simulink model "tqdtqr_rebuild_V3"  (R2021b)
settings: Solver=VariableStepAuto  StartTime=0.0  StopTime=10.0  RelTol=1e-3
undefined symbols (not defined in the file): ATQD_AfterTqMinGain_X_Deg, ATQD_APSCreepBaseTqD_X_kph, ATQD_APSCreepBaseTqD_Y_Deg, ATQD_APSCreepBaseTqR_X_kph, ATQD_APSCreepBaseTqR_Y_Deg, ATQD_APSCreepIterm_X_kph, ATQD_APSCreepIterm_Y_kph, ATQD_APSCreepPterm_X_kph, ATQD_APSCreepPterm_Y_kph, ATQD_APSDecReq_X_kph, ATQD_APSDecReq_Y_mps2, ATQD_APSDecReqCMD_X_kph, ATQD_APSDecReqTs_X_pct, ATQD_APSDecTimeGain_X_Deg, ATQD_APSDecTimeGain_Y_s, ATQD_APSReqLowSpd_X_Deg, ATQD_AutoHoldReleaseBPS_X_Deg, ATQD_AWDLoadTrqnsGain_X_kg, ATQD_AWDLoadTrqnsGain_Y_pct, ATQD_BOSEnBPSPosn_X_kph, ATQD_BOSMap_X_rpm, ATQD_BOSMap_Y_pct, ATQD_CreepBaseTqD_X_kph, ATQD_CreepBaseTqD_Y_Deg, ATQD_CreepBaseTqR_X_kph, ATQD_CreepBaseTqR_Y_Deg, ATQD_CreepBPSDisPosn_X_Deg, ATQD_CreepBPSDisPosnR_X_Deg, ATQD_CreepBPSEnPosn_X_Deg, ATQD_CreepBPSEnPosnR_X_Deg, ATQD_CreepDeltaTq_X_kph, ATQD_CreepIterm_X_kph, ATQD_CreepIterm_Y_kph, ATQD_CreepItermMaxLimit_X_pct, ATQD_CreepPreloadTime_X_kph, ATQD_CreepPreloadTq_X_kph, ATQD_CreepPreloadTq_Y_s, ATQD_CreepProtTq_X_Deg, ATQD_CreepPterm_X_kph, ATQD_CreepPterm_Y_kph, ATQD_CreepRrTqSpRat_X_rpm, ATQD_CreepRrTqSpRat_Y_Nm, ATQD_CreepTargetSpdD_X_pct, ATQD_CreepTargetSpdR_X_pct, ATQD_CreepUpLimitTq_X_rpm, ATQD_DecIneOPDHoldEnDelay_X_Deg, ATQD_DecIneOPDHoldEnDelay_Y_bar, ATQD_ECOTqMapD_X_rpm, ATQD_ECOTqMapD_Y_pct, ATQD_EMTqMapD_X_rpm, ATQD_EMTqMapD_Y_pct, ATQD_EOPDTqMapDCon_X_rpm, ATQD_EOPDTqMapDCon_Y_Deg, ATQD_EstInitVehWeight_X_c, ATQD_FAfterTqCMDGain_X_rpm, ATQD_FAfterTqCMDGain_Y_pct, ATQD_ForceLowSpd_X_Deg, ATQD_ForcePLimitSpd_X_Deg, ATQD_FrLossMAPLowV_X_rpm, ATQD_FrLossMAPLowV_Y_Nm ... (+949)
libraries: simulink x235, hcu_lib x208, tqr x63, tqd x6
(part 37 of 37)

== stateflow chart tqdtqr_rebuild_V3/Input_Convert/Signal function/SWC1 SWC2 status/SWC_Subsystem/Speed Setting Mode/ACC Speed Setting ON/ACCSetSpd_Chart_W ==
  state ACCSetSpeed_W
    (default) -> (junction 431) : {VTQD_ACCSetSpd_kph = ZERO_FLOAT;
        |  VTQD_ACCSavedSetSpd_kph = ZERO_FLOAT;
        |  VTQD_UpDownDetCount_sec = ZERO_FLOAT;
        |  VTQD_StandbyOvrdDetEnd_flg = FALSE;}
    ACCSetSpeed_W -> (junction 538) [order 3]
    (junction 538) -> (junction 552) [order 1] : [VTQD_DistanceUnit_flg == VINP_Distanceunit_flg || VTQD_ACCSavedSetSpd_kph <= ONE_FLOAT]
    (junction 552) -> (junction 431) : {VTQD_ACCSetSpd_kph = min(KTQD_ACCActiveMetSpdHi_raw32, VTQD_ACCSavedSetSpd_kph);
        |  VTQD_ACCSavedSetSpd_kph = VTQD_ACCSetSpd_kph;}
    (junction 538) -> (junction 540) [order 2]
    (junction 550) -> (junction 552)
    (junction 431) -> (junction 432) : {VSCP_ActiveDown_flg = FALSE;
        |  VTQD_ActiveUp_flg = FALSE;
        |  VTQD_UpDownTimeCount_sec = ZERO_FLOAT;}
    (junction 540) -> (junction 542) [order 1] : [VINP_Distanceunit_flg == TRUE]
    (junction 540) -> (junction 636) [order 2] : {VTQD_ACCSavedSetSpd_kph = (VTQD_ACCSavedSetSpd_kph * MPH2KPH)}
    (junction 542) -> (junction 599) : {VTQD_ACCSavedSetSpd_kph = (VTQD_ACCSavedSetSpd_kph * KPH2MPH)}
    (junction 432) -> (junction 530) [order 1] : [VINP_ADASACCSta_enum == ENUM_ADASACCSTA_STANDBY ||...
        |  VINP_ADASACCSta_enum == ENUM_ADASACCSTA_OVERRIDE]
    (junction 530) -> (junction 433) [order 1] : [VTQD_SWCSetDownSta_flg == TRUE ||...
        |  VTQD_SWCResUpSta_flg == TRUE]
    (junction 433) -> (junction 419) [order 1] : [VTQD_SWCSetDownSta_flg == TRUE &&...
        |  VTQD_StandbyOvrdDetEnd_flg == FALSE &&...
        |  VTQD_AllowSetSpd_flg == TRUE]
    (junction 432) -> (junction 403) [order 2]
    (junction 530) -> (junction 533) [order 2] : {VTQD_StandbyOvrdDetEnd_flg = FALSE;
        |  VTQD_ACCSetSpd_kph = VTQD_ACCSavedSetSpd_kph;
        |  VTQD_ACCSavedSetSpd_kph = VTQD_ACCSetSpd_kph;
        |  VTQD_DistanceUnit_flg = VINP_Distanceunit_flg;}
    (junction 433) -> (junction 490) [order 2]
    (junction 419) -> (junction 408) : {VTQD_UpDownDetCount_sec = VTQD_UpDownDetCount_sec + task_time_s;}
    (junction 599) -> (junction 602) [order 1] : [VTQD_ACCSavedSetSpd_kph < KTQD_ACCActiveMetSpdLoMPH_mph]
    (junction 636) -> (junction 623) [order 1] : [VTQD_ACCSavedSetSpd_kph < KTQD_ACCActiveMetSpdLo_kph]
    (junction 602) -> (junction 604) : {VTQD_ACCSavedSetSpd_kph = KTQD_ACCActiveMetSpdLoMPH_mph}
    (junction 636) -> (junction 633) [order 2]
    (junction 623) -> (junction 619) : {VTQD_ACCSavedSetSpd_kph = KTQD_ACCActiveMetSpdLo_kph}
    (junction 599) -> (junction 606) [order 2]
    (junction 604) -> (junction 606)
    (junction 619) -> (junction 633)
    (junction 606) -> (junction 613)
    (junction 633) -> (junction 630)
    (junction 630) -> (junction 625) [order 1] : [VTQD_ACCSavedSetSpd_kph > KTQD_ACCActiveMetSpdHi_kph]
    (junction 613) -> (junction 608) [order 1] : [VTQD_ACCSavedSetSpd_kph > KTQD_ACCActiveMetSpdHiMPH_mph]
    (junction 403) -> (junction 395) [order 1] : [(VTQD_SWCSetDownSta_flg == TRUE ||...
        |   VTQD_SWCResUpSta_flg == TRUE) &&...
        |  (VTQD_StandbyOvrdDetEnd_flg == TRUE ||...
        |   VTQD_HoldResDet_flg == TRUE)]
    (junction 490) -> (junction 492) [order 1] : [VINP_ADASACCSta_enum == ENUM_ADASACCSTA_STANDBY &&...
        |  VTQD_SWCResUpSta_flg == TRUE &&...
        |  VTQD_ACCSavedSetSpd_kph > ZERO_FLOAT]
    (junction 408) -> (junction 409) [order 1] : [VTQD_UpDownDetCount_sec > ZERO_FLOAT]
    (junction 409) -> (junction 405) [order 1] : [KTQD_ACCActiveMetSpdHi_raw32 >= VVMC_MeterIndSpeed_raw32 &&...
        |  VVMC_MeterIndSpeed_raw32 >= KTQD_ACCActiveMetSpdLo_raw32]
    (junction 630) -> (junction 632) [order 2]
    (junction 625) -> (junction 628) : {VTQD_ACCSavedSetSpd_kph = KTQD_ACCActiveMetSpdHi_kph}
    (junction 613) -> (junction 615) [order 2]
    (junction 608) -> (junction 612) : {VTQD_ACCSavedSetSpd_kph = KTQD_ACCActiveMetSpdHiMPH_mph}
    (junction 403) -> (junction 396) [order 2] : {VTQD_StandbyOvrdDetEnd_flg = FALSE;
        |  VTQD_HoldResDet_flg = FALSE;}
    (junction 395) -> (junction 399) : {VTQD_StandbyOvrdDetEnd_flg = TRUE;
        |  VTQD_HoldResDet_flg = TRUE;}
    (junction 490) -> (junction 496) [order 2]
    (junction 492) -> (junction 494) : {VTQD_StandbyOvrdDetEnd_flg = TRUE}
    (junction 408) -> (junction 436) [order 2] : {VTQD_ACCSetSpd_kph = VTQD_ACCSavedSetSpd_kph;
        |  VTQD_ACCSavedSetSpd_kph = VTQD_ACCSetSpd_kph;
        |  VTQD_DistanceUnit_flg = VINP_Distanceunit_flg;}
    (junction 409) -> (junction 410) [order 2]
    (junction 405) -> (junction 435) : {VTQD_ACCSetSpd_kph = VVMC_MeterIndSpeed_raw32;
        |  VTQD_ACCSavedSetSpd_kph = VTQD_ACCSetSpd_kph;
        |  VTQD_StandbyOvrdDetEnd_flg = TRUE;
        |  VTQD_UpDownDetCount_sec = ZERO_FLOAT;
        |  VTQD_DistanceUnit_flg = VINP_Distanceunit_flg;}
    (junction 628) -> (junction 632)
    (junction 612) -> (junction 615)
    (junction 632) -> (junction 547)
    (junction 615) -> (junction 544)
    (junction 547) -> (junction 544)
    (junction 544) -> (junction 550)
    (junction 494) -> (junction 496)
    (junction 410) -> (junction 429) [order 1] : [KTQD_ACCActiveMetSpdHi_raw32 < VVMC_MeterIndSpeed_raw32]
    (junction 496) -> (junction 407) : {VTQD_ACCSetSpd_kph = VTQD_ACCSavedSetSpd_kph;
        |  VTQD_ACCSavedSetSpd_kph = VTQD_ACCSetSpd_kph;
        |  VTQD_DistanceUnit_flg = VINP_Distanceunit_flg;}
    (junction 410) -> (junction 420) [order 2] : {VTQD_ACCSetSpd_kph = KTQD_ACCActiveMetSpdLo_raw32;
        |  VTQD_ACCSavedSetSpd_kph = VTQD_ACCSetSpd_kph;
        |  VTQD_StandbyOvrdDetEnd_flg = TRUE;
        |  VTQD_UpDownDetCount_sec = ZERO_FLOAT;
        |  VTQD_DistanceUnit_flg = VINP_Distanceunit_flg;}
    (junction 429) -> (junction 430) : {VTQD_ACCSetSpd_kph = KTQD_ACCActiveMetSpdHi_raw32;
        |  VTQD_ACCSavedSetSpd_kph = VTQD_ACCSetSpd_kph;
        |  VTQD_StandbyOvrdDetEnd_flg = TRUE;
        |  VTQD_UpDownDetCount_sec = ZERO_FLOAT;
        |  VTQD_DistanceUnit_flg = VINP_Distanceunit_flg;}
    (junction 399) -> (junction 396)
    (junction 396) -> (junction 438)
    (junction 438) -> (junction 417) [order 1] : [VINP_ADASACCSta_enum == ENUM_ADASACCSTA_ACTIVE]
    (junction 417) -> (junction 434) [order 1] : [VTQD_SWCSetDownSta_flg == TRUE &&...
        |  VTQD_StandbyOvrdDetEnd_flg == FALSE &&...
        |  VVMC_LVDAACCStatusInformation_flg == FALSE]
    (junction 438) -> (junction 427) [order 2]
    (junction 417) -> (junction 412) [order 2]
    (junction 434) -> (junction 411) : {VTQD_UpDownDetCount_sec = VTQD_UpDownDetCount_sec + task_time_s;}
    (junction 411) -> (junction 437) [order 1] : [VTQD_UpDownDetCount_sec > ZERO_FLOAT]
    (junction 411) -> (junction 406) [order 2] : {VTQD_ACCSetSpd_kph = VTQD_ACCSavedSetSpd_kph;
        |  VTQD_ACCSavedSetSpd_kph = VTQD_ACCSetSpd_kph;
        |  VTQD_DistanceUnit_flg = VINP_Distanceunit_flg;}
    (junction 437) -> (junction 428) : {VTQD_ACCSetSpd_kph = max(KTQD_ACCActiveMetSpdLo_raw32, VTQD_ACCSavedSetSpd_kph - ONE_FLOAT);
        |  VTQD_ACCSavedSetSpd_kph = VTQD_ACCSetSpd_kph;
        |  VSCP_ActiveDown_flg = TRUE;
        |  VTQD_UpDownDetCount_sec = ZERO_FLOAT;
        |  VTQD_UpDownTimeCount_sec = task_time_s;
        |  VTQD_DistanceUnit_flg = VINP_Distanceunit_flg;}
    (junction 427) -> (junction 404) [order 1] : [VINP_ADASACCSta_enum == ENUM_ADASACCSTA_OFF ||...
        |  VINP_ADASACCSta_enum == ENUM_ADASACCSTA_DISABLE||...
        |  VINP_ADASACCSta_enum == ENUM_ADASACCSTA_ERROR]
    (junction 412) -> (junction 510) [order 1] : [VTQD_SWCResUpSta_flg == TRUE]
    (junction 510) -> (junction 413) [order 1] : [VTQD_StandbyOvrdDetEnd_flg == FALSE &&...
        |  VVMC_LVDAACCStatusInformation_flg == FALSE &&...
        |  VTQD_HoldResDet_flg == FALSE]
    (junction 427) -> (junction 422) [order 2] : {VTQD_ACCSetSpd_kph = VTQD_ACCSavedSetSpd_kph;
        |  VTQD_ACCSavedSetSpd_kph = VTQD_ACCSetSpd_kph;
        |  VTQD_DistanceUnit_flg = VINP_Distanceunit_flg;}
    (junction 404) -> (junction 426) : {VTQD_ACCSetSpd_kph = ZERO_FLOAT;
        |  VTQD_ACCSavedSetSpd_kph = VTQD_ACCSetSpd_kph;
        |  VTQD_DistanceUnit_flg = VINP_Distanceunit_flg;}
    (junction 412) -> (junction 522) [order 2]
    (junction 510) -> (junction 512) [order 2]
    (junction 413) -> (junction 414) : {VTQD_UpDownDetCount_sec = VTQD_UpDownDetCount_sec + task_time_s;}
    (junction 512) -> (junction 514) [order 1] : [VTQD_StandbyOvrdDetEnd_flg == FALSE &&...
        |  VVMC_LVDAACCStatusInformation_flg != FALSE]
    (junction 414) -> (junction 415) [order 1] : [VTQD_UpDownDetCount_sec > ZERO_FLOAT]
    (junction 512) -> (junction 519) [order 2]
    (junction 514) -> (junction 516) : {VTQD_HoldResDet_flg = TRUE}
    (junction 414) -> (junction 418) [order 2] : {VTQD_ACCSetSpd_kph = VTQD_ACCSavedSetSpd_kph;
        |  VTQD_ACCSavedSetSpd_kph = VTQD_ACCSetSpd_kph;
        |  VTQD_DistanceUnit_flg = VINP_Distanceunit_flg;}
    (junction 415) -> (junction 421) : {VTQD_ACCSetSpd_kph = min(KTQD_ACCActiveMetSpdHi_raw32, VTQD_ACCSavedSetSpd_kph + ONE_FLOAT);
        |  VTQD_ACCSavedSetSpd_kph = VTQD_ACCSetSpd_kph;
        |  VTQD_ActiveUp_flg = TRUE;
        |  VTQD_UpDownDetCount_sec = ZERO_FLOAT;
        |  VTQD_UpDownTimeCount_sec = task_time_s;
        |  VTQD_DistanceUnit_flg = VINP_Distanceunit_flg;}
    (junction 519) -> (junction 522)
    (junction 516) -> (junction 519)
    (junction 522) -> (junction 416) : {VTQD_ACCSetSpd_kph = VTQD_ACCSavedSetSpd_kph;
        |  VTQD_ACCSavedSetSpd_kph = VTQD_ACCSetSpd_kph;
        |  VTQD_DistanceUnit_flg = VINP_Distanceunit_flg;}
    ACCSetSpeed_W -> (junction 568) [order 1] : [VSCP_ActiveDown_flg == TRUE &&...
        |  VINP_ADASACCSta_enum == ENUM_ADASACCSTA_ACTIVE &&...
        |  VTQD_SWCSetDownSta_flg == TRUE]
    (junction 568) -> (junction 556) [order 1] : [VTQD_DistanceUnit_flg == VINP_Distanceunit_flg]
    (junction 556) -> (junction 423)
    (junction 568) -> (junction 558) [order 2]
    (junction 560) -> (junction 556)
    (junction 423) -> (junction 424) : {VTQD_UpDownTimeCount_sec = VTQD_UpDownTimeCount_sec + task_time_s}
    (junction 558) -> (junction 566) [order 1] : [VINP_Distanceunit_flg == TRUE]
    (junction 558) -> (junction 571) [order 2] : {VTQD_ACCSavedSetSpd_kph = (VTQD_ACCSavedSetSpd_kph * MPH2KPH)}
    (junction 566) -> (junction 557) : {VTQD_ACCSavedSetSpd_kph = (VTQD_ACCSavedSetSpd_kph * KPH2MPH)}
    (junction 424) -> (junction 466) [order 1] : [VTQD_UpDownTimeCount_sec >= KTQD_SetSpdLongPLim_s]
    (junction 424) -> (junction 444) [order 2] : {VTQD_ACCSetSpd_kph = VTQD_ACCSavedSetSpd_kph;
        |  VTQD_ACCSavedSetSpd_kph = VTQD_ACCSetSpd_kph;
        |  VTQD_DistanceUnit_flg = VINP_Distanceunit_flg;}
    (junction 466) -> (junction 478) : {VTQD_ACCSetSpd_kph = max(KTQD_ACCActiveMetSpdLo_raw32, ceil(VTQD_ACCSavedSetSpd_kph / KTQD_SetSpdDeltaLong_kph - ONE_FLOAT) * KTQD_SetSpdDeltaLong_kph);
        |  VTQD_ACCSavedSetSpd_kph = VTQD_ACCSetSpd_kph;
        |  VTQD_UpDownTimeCount_sec = ZERO_FLOAT;
        |  VTQD_DistanceUnit_flg = VINP_Distanceunit_flg;}
    (junction 571) -> (junction 557)
    (junction 557) -> (junction 560)
    ACCSetSpeed_W -> (junction 585) [order 2] : [VTQD_ActiveUp_flg == TRUE &&...
        |  VINP_ADASACCSta_enum == ENUM_ADASACCSTA_ACTIVE &&...
        |  VTQD_SWCResUpSta_flg == TRUE]
    (junction 585) -> (junction 583) [order 1] : [VTQD_DistanceUnit_flg == VINP_Distanceunit_flg]
    (junction 583) -> (junction 479)
    (junction 585) -> (junction 584) [order 2]
    (junction 580) -> (junction 583)
    (junction 479) -> (junction 480) : {VTQD_UpDownTimeCount_sec = VTQD_UpDownTimeCount_sec + task_time_s}
    (junction 584) -> (junction 576) [order 1] : [VINP_Distanceunit_flg == TRUE]
    (junction 584) -> (junction 573) [order 2] : {VTQD_ACCSavedSetSpd_kph = (VTQD_ACCSavedSetSpd_kph * MPH2KPH)}
    (junction 576) -> (junction 582) : {VTQD_ACCSavedSetSpd_kph = (VTQD_ACCSavedSetSpd_kph * KPH2MPH)}
    (junction 480) -> (junction 463) [order 1] : [VTQD_UpDownTimeCount_sec >= KTQD_SetSpdLongPLim_s]
    (junction 480) -> (junction 455) [order 2] : {VTQD_ACCSetSpd_kph = VTQD_ACCSavedSetSpd_kph;
        |  VTQD_ACCSavedSetSpd_kph = VTQD_ACCSetSpd_kph;
        |  VTQD_DistanceUnit_flg = VINP_Distanceunit_flg;}
    (junction 463) -> (junction 461) : {VTQD_ACCSetSpd_kph = min(KTQD_ACCActiveMetSpdHi_raw32, floor(VTQD_ACCSavedSetSpd_kph / KTQD_SetSpdDeltaLong_kph + ONE_FLOAT) * KTQD_SetSpdDeltaLong_kph);
        |  VTQD_ACCSavedSetSpd_kph = VTQD_ACCSetSpd_kph;
        |  VTQD_UpDownTimeCount_sec = ZERO_FLOAT;
        |  VTQD_DistanceUnit_flg = VINP_Distanceunit_flg;}
    (junction 573) -> (junction 582)
    (junction 582) -> (junction 580)
  data: VINP_ADASACCSta_enum input uint8; VTQD_SWCResUpSta_flg input boolean; VTQD_SWCSetDownSta_flg input boolean; VVMC_MeterIndSpeed_raw32 input single; KTQD_ACCActiveMetSpdHi_raw32 input uint8; VINP_Distanceunit_flg input boolean; KTQD_ACCActiveMetSpdLo_raw32 input uint8; VTQD_ACCSetSpd_kph output single; KTQD_SetSpdDeltaLong_kph input uint8; VTQD_ACCSavedSetSpd_kph local single; ENUM_ADASACCSTA_STANDBY parameter uint8; ZERO_FLOAT parameter single; TRUE parameter boolean; ENUM_ADASACCSTA_ACTIVE parameter uint8; ONE_FLOAT parameter single; FALSE parameter boolean; VSCP_ActiveDown_flg local boolean; VTQD_UpDownTimeCount_sec local single; VTQD_ActiveUp_flg local boolean; KTQD_SetSpdLongPLim_s input single; VTQD_UpDownDetCount_sec local single; ENUM_ADASACCSTA_OVERRIDE parameter uint8; VTQD_StandbyOvrdDetEnd_flg local boolean; ENUM_ADASACCSTA_DISABLE parameter; ENUM_ADASACCSTA_OFF parameter; ENUM_ADASACCSTA_ERROR parameter; VVMC_LVDAACCStatusInformation_flg input; VTQD_HoldResDet_flg local boolean; VTQD_AllowSetSpd_flg input; task_time_s input; VTQD_DistanceUnit_flg local boolean; KPH2MPH parameter; MPH2KPH parameter; KTQD_ACCActiveMetSpdLo_kph parameter; KTQD_ACCActiveMetSpdLoMPH_mph parameter; KTQD_ACCActiveMetSpdHiMPH_mph parameter; KTQD_ACCActiveMetSpdHi_kph parameter

== stateflow chart tqdtqr_rebuild_V3/Input_Convert/Signal function/SWC1 SWC2 status/SWC_Subsystem/Speed Setting Mode/CC Speed Setting ON/CC Speed Setting Mode ==
  state CC
    en:
    VTQD_CCSetSpd_kph = 0;
    VTQD_CCSavedSetSpd_kph = 0;
    VTQD_CCSpdResetFinish_flg = 0;
    state Active
      (default) -> (junction 61)
      (junction 61) -> (junction 65) [order 1] : [VTQD_SWCResUpPress_enum == ENUM_SWCBOTTONPRESS_LONGPRESS  ||...
          |  VTQD_SWCResUpPress_enum == ENUM_SWCBOTTONPRESS_SHORTPRESS ||...
          | VTQD_SWCSetDownPress_enum == ENUM_SWCBOTTONPRESS_LONGPRESS  ||...
          |  VTQD_SWCSetDownPress_enum == ENUM_SWCBOTTONPRESS_SHORTPRESS   ]
      (junction 65) -> (junction 69) [order 1] : [VTQD_SWCSetDownPress_enum == ENUM_SWCBOTTONPRESS_LONGPRESS  ||...
          |  VTQD_SWCSetDownPress_enum == ENUM_SWCBOTTONPRESS_SHORTPRESS ]
      (junction 61) -> (junction 63) [order 2]
      (junction 65) -> (junction 67) [order 2]
      (junction 69) -> (junction 80)
      (junction 67) -> (junction 71) [order 1] : [VTQD_SWCResUpPress_enum == ENUM_SWCBOTTONPRESS_LONGPRESS]
      (junction 80) -> (junction 82) [order 1] : [VTQD_SWCSetDownPress_enum == ENUM_SWCBOTTONPRESS_LONGPRESS]
      (junction 67) -> (junction 73) [order 2] : %ADD_Short
          | {VTQD_CCSetSpd_kph = VTQD_CCSetSpd_kph + KTQD_SetSpdDeltaShort_kph; ...
          | VTQD_CCSetSpd_kph = min (KTQD_CCActiveMetSpdHi_raw32,VTQD_CCSetSpd_kph);...
          | VTQD_CCSavedSetSpd_kph = VTQD_CCSetSpd_kph;
          | VTQD_DistanceUnit_flg = VINP_Distanceunit_flg
          | }
      (junction 80) -> (junction 83) [order 2] : %SUBSTRACT_Short
          | {VTQD_CCSetSpd_kph = VTQD_CCSetSpd_kph - KTQD_SetSpdDeltaShort_kph; ...
          | VTQD_CCSetSpd_kph = max (KTQD_CCActiveMetSpdLo_raw32,VTQD_CCSetSpd_kph);...
          | VTQD_CCSavedSetSpd_kph = VTQD_CCSetSpd_kph;
          | VTQD_DistanceUnit_flg = VINP_Distanceunit_flg
          | }
      (junction 71) -> (junction 272)
      (junction 82) -> (junction 278)
      (junction 272) -> (junction 274) [order 1] : [VTQD_SetSpdDeltaLongFit_kph != 0]
      (junction 278) -> (junction 282) [order 1] : [VTQD_SetSpdDeltaLongFit_kph != 0]
      (junction 272) -> (junction 75) [order 2] : %ADD_Long
          | {VTQD_CCSetSpd_kph = VTQD_CCSetSpd_kph + KTQD_SetSpdDeltaLong_kph; ...
          | VTQD_CCSetSpd_kph = min (KTQD_CCActiveMetSpdHi_raw32,VTQD_CCSetSpd_kph);...
          | VTQD_CCSavedSetSpd_kph = VTQD_CCSetSpd_kph;
          | VTQD_DistanceUnit_flg = VINP_Distanceunit_flg
          | }
      (junction 274) -> (junction 276) : {
          | VTQD_CCSetSpd_kph = VTQD_CCSetSpd_kph + (KTQD_SetSpdDeltaLongFit_kph-VTQD_SetSpdDeltaLongFit_kph); ...
          | VTQD_CCSetSpd_kph = min (KTQD_CCActiveMetSpdHi_raw32,VTQD_CCSetSpd_kph); ...
          | VTQD_CCSavedSetSpd_kph = VTQD_CCSetSpd_kph;
          | VTQD_DistanceUnit_flg = VINP_Distanceunit_flg
          | }
          | %add20231127
      (junction 278) -> (junction 85) [order 2] : %SUBSTRACT_Long
          | {VTQD_CCSetSpd_kph = VTQD_CCSetSpd_kph - KTQD_SetSpdDeltaLong_kph; ...
          | VTQD_CCSetSpd_kph = max (KTQD_CCActiveMetSpdLo_raw32,VTQD_CCSetSpd_kph);...
          | VTQD_CCSavedSetSpd_kph = VTQD_CCSetSpd_kph;
          | VTQD_DistanceUnit_flg = VINP_Distanceunit_flg
          | }
      (junction 282) -> (junction 284) : {VTQD_CCSetSpd_kph = VTQD_CCSetSpd_kph - VTQD_SetSpdDeltaLongFit_kph; ...
          | VTQD_CCSetSpd_kph = max (KTQD_CCActiveMetSpdLo_raw32,VTQD_CCSetSpd_kph);...
          | VTQD_CCSavedSetSpd_kph = VTQD_CCSetSpd_kph;
          | VTQD_DistanceUnit_flg = VINP_Distanceunit_flg}
          | %add20231122
    state OFForDisable
      en:
      VTQD_CCSetSpd_kph = 0;
      VTQD_CCSavedSetSpd_kph=VTQD_CCSetSpd_kph;
      VTQD_DistanceUnit_flg = VINP_Distanceunit_flg
    state ChangeFrom_ACTIVE
      (default) -> (junction 238)
      (junction 238) -> (junction 239) [order 1] : [VTQD_CCSpdResetFinish_flg]
      (junction 238) -> (junction 241) [order 2] : {VTQD_CCSetSpd_kph = VTQD_CCSavedSetSpd_kph;}
          | %add20231206
      (junction 239) -> (junction 244)
      (junction 244) -> (junction 241)
      (junction 241) -> (junction 206)
      (junction 206) -> (junction 203) [order 1] : [VTQD_SWCResUpPress_enum == ENUM_SWCBOTTONPRESS_LONGPRESS  ||...
          |  VTQD_SWCResUpPress_enum == ENUM_SWCBOTTONPRESS_SHORTPRESS ||...
          | VTQD_SWCSetDownPress_enum == ENUM_SWCBOTTONPRESS_LONGPRESS  ||...
          |  VTQD_SWCSetDownPress_enum == ENUM_SWCBOTTONPRESS_SHORTPRESS   ]
      (junction 203) -> (junction 205) [order 1] : [VTQD_SWCResUpPress_enum == ENUM_SWCBOTTONPRESS_LONGPRESS  ||...
          |  VTQD_SWCResUpPress_enum == ENUM_SWCBOTTONPRESS_SHORTPRESS ]
      (junction 203) -> (junction 209) [order 2] : {VTQD_CCSetSpd_kph = VVMC_MeterIndSpeed_raw32;
          | VTQD_CCSpdResetFinish_flg = TRUE;
          | VTQD_CCSetSpd_kph = max (KTQD_CCActiveMetSpdLo_raw32,VTQD_CCSetSpd_kph);
          | VTQD_CCSavedSetSpd_kph=VTQD_CCSetSpd_kph;
          | VTQD_DistanceUnit_flg = VINP_Distanceunit_flg}
          | %add20231206
      (junction 206) -> (junction 211) [order 2]
      (junction 205) -> (junction 210) : {VTQD_CCSetSpd_kph = VTQD_CCSavedSetSpd_kph;
          | VTQD_CCSpdResetFinish_flg = TRUE;
          | VTQD_CCSavedSetSpd_kph=VTQD_CCSetSpd_kph;
          | VTQD_DistanceUnit_flg = VINP_Distanceunit_flg}
    state SetDown
    state LoopBack
    (default) -> (junction 1) : {VTQD_DistanceUnit_flg = VINP_Distanceunit_flg}
    (junction 253) -> (junction 258) [order 2]
    (junction 258) -> (junction 300)
    (junction 300) -> (junction 290) [order 1] : [VTQD_DistanceUnit_flg == VINP_Distanceunit_flg || VTQD_CCSavedSetSpd_kph <= ONE_FLOAT]
    CC -> (junction 253)
    (junction 290) -> (junction 1) : {VTQD_CCSetSpd_kph = min (KTQD_CCActiveMetSpdHi_raw32,VTQD_CCSetSpd_kph);
        | VTQD_CCSavedSetSpd_kph = VTQD_CCSetSpd_kph;}
    (junction 1) -> (junction 3) [order 1] : [VVMC_CCCtrlSta_enum != ENUM_ADASCCSTA_STANDBY &&...
        |  VVMC_CCCtrlSta_enum != ENUM_ADASCCSTA_ACTIVE &&...
        |  VVMC_CCCtrlSta_enum != ENUM_ADASCCSTA_OVRRIDE]
    (junction 300) -> (junction 289) [order 2]
    (junction 253) -> (junction 255) [order 1]
    (junction 256) -> (junction 258) : {VTQD_CCSpdResetFinish_flg = FALSE;}
    (junction 292) -> (junction 290)
    (junction 1) -> (junction 20) [order 2]
    (junction 3) -> OFForDisable
    (junction 289) -> (junction 295) [order 1] : [VINP_Distanceunit_flg == TRUE]
    (junction 289) -> (junction 340) [order 2] : {VTQD_CCSavedSetSpd_kph = (VTQD_CCSavedSetSpd_kph * MPH2KPH)}
    (junction 295) -> (junction 342) : {VTQD_CCSavedSetSpd_kph = (VTQD_CCSavedSetSpd_kph * KPH2MPH)}
    (junction 255) -> (junction 256) : [VVMC_CCCtrlSta_enum != ENUM_ADASCCSTA_STANDBY &&...
        | VTQD_CCSpdResetFinish_flg]
    (junction 20) -> (junction 228) [order 1] : [VVMC_CCCtrlSta_enum == ENUM_ADASCCSTA_ACTIVE ||...
        | VVMC_CCCtrlSta_enum == ENUM_ADASCCSTA_OVRRIDE
        | ]
    (junction 228) -> (junction 25) [order 2]
    (junction 20) -> (junction 181) [order 2]
    (junction 228) -> (junction 28) [order 1] : [VVMC_CCCtrlSta_enum == ENUM_ADASCCSTA_OVRRIDE]
    (junction 25) -> Active : {VTQD_CCSetSpd_kph = VTQD_CCSavedSetSpd_kph;
        | VTQD_CCSavedSetSpd_kph=VTQD_CCSetSpd_kph;
        | VTQD_DistanceUnit_flg = VINP_Distanceunit_flg}
    (junction 340) -> (junction 323) [order 1] : [VTQD_CCSavedSetSpd_kph < KTQD_CCActiveMetSpdLo_kph]
    (junction 342) -> (junction 311) [order 1] : [VTQD_CCSavedSetSpd_kph < KTQD_CCActiveMetSpdLoMPH_mph]
    (junction 340) -> (junction 324) [order 2]
    (junction 323) -> (junction 326) : {VTQD_CCSavedSetSpd_kph = KTQD_CCActiveMetSpdLo_kph}
    (junction 342) -> (junction 321) [order 2]
    (junction 311) -> (junction 307) : {VTQD_CCSavedSetSpd_kph = KTQD_CCActiveMetSpdLoMPH_mph}
    (junction 181) -> (junction 28) [order 1] : [VVMC_CCCtrlSta_enum == ENUM_ADASCCSTA_STANDBY]
    (junction 28) -> (junction 40) [order 1] : [VTQD_ChangeToSTANDBY_flg]
    (junction 181) -> LoopBack [order 2] : {VTQD_CCSetSpd_kph = VTQD_CCSavedSetSpd_kph;
        | VTQD_CCSavedSetSpd_kph=VTQD_CCSetSpd_kph;
        | VTQD_DistanceUnit_flg = VINP_Distanceunit_flg}
    (junction 28) -> (junction 43) [order 2]
    (junction 40) -> ChangeFrom_ACTIVE : {VTQD_CCSetSpd_kph = VTQD_CCSavedSetSpd_kph;
        | VTQD_CCSavedSetSpd_kph=VTQD_CCSetSpd_kph;
        | VTQD_DistanceUnit_flg = VINP_Distanceunit_flg}
    (junction 307) -> (junction 321)
    (junction 326) -> (junction 324)
    (junction 321) -> (junction 318)
    (junction 324) -> (junction 330)
    (junction 330) -> (junction 328) [order 1] : [VTQD_CCSavedSetSpd_kph > KTQD_CCActiveMetSpdHi_kph]
    (junction 318) -> (junction 313) [order 1] : [VTQD_CCSavedSetSpd_kph > KTQD_CCActiveMetSpdHiMPH_mph]
    (junction 330) -> (junction 334) [order 2]
    (junction 328) -> (junction 331) : {VTQD_CCSavedSetSpd_kph = KTQD_CCActiveMetSpdHi_kph}
    (junction 318) -> (junction 320) [order 2]
    (junction 313) -> (junction 316) : {VTQD_CCSavedSetSpd_kph = KTQD_CCActiveMetSpdHiMPH_mph}
    (junction 43) -> (junction 44) [order 1] : [VTQD_SWCSetDownPress_enum == ENUM_SWCBOTTONPRESS_LONGPRESS  ||...
        |  VTQD_SWCSetDownPress_enum == ENUM_SWCBOTTONPRESS_SHORTPRESS ]
    (junction 43) -> LoopBack [order 2] : {VTQD_CCSetSpd_kph = VTQD_CCSavedSetSpd_kph;
        | VTQD_CCSavedSetSpd_kph=VTQD_CCSetSpd_kph;
        | VTQD_DistanceUnit_flg = VINP_Distanceunit_flg}
    (junction 44) -> SetDown : {VTQD_CCSetSpd_kph = VVMC_MeterIndSpeed_raw32;
        | VTQD_CCSetSpd_kph = max (KTQD_CCActiveMetSpdLo_raw32,VTQD_CCSetSpd_kph);
        | VTQD_CCSavedSetSpd_kph=VTQD_CCSetSpd_kph;
        | VTQD_DistanceUnit_flg = VINP_Distanceunit_flg}
        | %add20231201
    (junction 331) -> (junction 334)
    (junction 316) -> (junction 320)
    (junction 334) -> (junction 301)
    (junction 320) -> (junction 291)
    (junction 301) -> (junction 291)
    (junction 291) -> (junction 292)
  data: KTQD_SetSpdDeltaLong_kph input; KTQD_SetSpdDeltaShort_kph input; KTQD_SetSpdDeltaLongFit_kph input; VTQD_SetSpdDeltaLongFit_kph input; VVMC_CCCtrlSta_enum input; VINP_Distanceunit_flg input; KTQD_CCActiveMetSpdHi_raw32 input; KTQD_CCActiveMetSpdLo_raw32 input; VVMC_MeterIndSpeed_raw32 input; VTQD_CCSetSpd_kph output single; VTQD_CCSavedSetSpd_kph local single; ENUM_ADASCCSTA_ACTIVE parameter; ENUM_ADASCCSTA_STANDBY parameter; VTQD_SWCSetDownPress_enum input; VTQD_SWCResUpPress_enum input; VTQD_ChangeToSTANDBY_flg input; ENUM_ADASCCSTA_OVRRIDE parameter; VTQD_CCSpdResetFinish_flg output; ENUM_SWCBOTTONPRESS_LONGPRESS parameter; ENUM_SWCBOTTONPRESS_SHORTPRESS parameter; FALSE parameter; TRUE parameter; KPH2MPH parameter; MPH2KPH parameter; VTQD_DistanceUnit_flg local boolean; ONE_FLOAT parameter; KTQD_CCActiveMetSpdHiMPH_mph parameter; KTQD_CCActiveMetSpdHi_kph parameter; KTQD_CCActiveMetSpdLoMPH_mph parameter; KTQD_CCActiveMetSpdLo_kph parameter

== stateflow chart tqdtqr_rebuild_V3/Input_Convert/Signal function/SWC1 SWC2 status/SWC_Subsystem/Speed Setting Mode/CC Speed Setting ON/Specific_STATE_ChangeToSTANDBY ==
  state FLG_ON
    en:
    VTQD_CCChangeToSTANDBY_flg = TRUE;
  state Initialize
    en:
    VTQD_CCChangeToSTANDBY_flg = FALSE;
  state STAY
  (default) -> Initialize
  Initialize -> STAY : [VVMC_CCCtrlSta_enum == ENUM_ADASCCSTA_ACTIVE]
  STAY -> FLG_ON [order 1] : [VVMC_CCCtrlSta_enum == ENUM_ADASCCSTA_STANDBY]
  STAY -> Initialize [order 2] : [VVMC_CCCtrlSta_enum != ENUM_ADASCCSTA_ACTIVE &&...
      | VVMC_CCCtrlSta_enum != ENUM_ADASCCSTA_STANDBY ]
  (junction 11) -> Initialize
  FLG_ON -> (junction 9)
  (junction 9) -> (junction 11) : [VVMC_CCCtrlSta_enum != ENUM_ADASCCSTA_STANDBY]
  data: VVMC_CCCtrlSta_enum input; FALSE parameter; TRUE parameter; VTQD_CCChangeToSTANDBY_flg output boolean; ENUM_ADASCCSTA_ACTIVE parameter; ENUM_ADASCCSTA_STANDBY parameter

== stateflow chart tqdtqr_rebuild_V3/Input_Convert/Signal function/SWC1 SWC2 status/SWC_Subsystem/Speed Setting Mode/MSA Speed Setting ON/MSA ==
  state MSA
    en:
    VTQD_MSASetSpd_kph = 0;
    VTQD_MSASavedSetSpd_kph = 0;
    state Active
      (default) -> (junction 219)
      (junction 219) -> (junction 220) [order 1] : [VTQD_SWCResUpPress_enum == ENUM_SWCBOTTONPRESS_LONGPRESS  ||...
          |  VTQD_SWCResUpPress_enum == ENUM_SWCBOTTONPRESS_SHORTPRESS ||...
          | VTQD_SWCSetDownPress_enum == ENUM_SWCBOTTONPRESS_LONGPRESS  ||...
          |  VTQD_SWCSetDownPress_enum == ENUM_SWCBOTTONPRESS_SHORTPRESS ]
      (junction 220) -> (junction 221) [order 1] : [VTQD_SWCSetDownPress_enum == ENUM_SWCBOTTONPRESS_LONGPRESS  ||...
          |  VTQD_SWCSetDownPress_enum == ENUM_SWCBOTTONPRESS_SHORTPRESS]
      (junction 219) -> (junction 226) [order 2]
      (junction 220) -> (junction 222) [order 2]
      (junction 221) -> (junction 224)
      (junction 222) -> (junction 223) [order 1] : [VTQD_SWCResUpPress_enum == ENUM_SWCBOTTONPRESS_LONGPRESS]
      (junction 224) -> (junction 225) [order 1] : [VTQD_SWCSetDownPress_enum == ENUM_SWCBOTTONPRESS_LONGPRESS]
      (junction 222) -> (junction 227) [order 2] : %ADD_Short
          | {VTQD_MSASetSpd_kph = VTQD_MSASetSpd_kph + KTQD_SetSpdDeltaShort_kph; ...
          | VTQD_MSASetSpd_kph = min (KTQD_MSAActiveMetSpdHi_raw32,VTQD_MSASetSpd_kph);...
          | VTQD_MSASavedSetSpd_kph = VTQD_MSASetSpd_kph;
          | VTQD_DistanceUnit_flg = VINP_Distanceunit_flg
          | %add20230704
          | }
      (junction 224) -> (junction 229) [order 2] : %SUBSTRACT_Short
          | {VTQD_MSASetSpd_kph = VTQD_MSASetSpd_kph - KTQD_SetSpdDeltaShort_kph; ...
          | VTQD_MSASetSpd_kph = max (KTQD_MSAActiveMetSpdLo_raw32,VTQD_MSASetSpd_kph);...
          | VTQD_MSASavedSetSpd_kph = VTQD_MSASetSpd_kph;
          | VTQD_DistanceUnit_flg = VINP_Distanceunit_flg
          | }
      (junction 223) -> (junction 289)
      (junction 225) -> (junction 296)
      (junction 296) -> (junction 298) [order 1] : [VTQD_SetSpdDeltaLongFit_kph  != 0]
      (junction 296) -> (junction 230) [order 2] : %SUBSTRACT_Long
          | {VTQD_MSASetSpd_kph = VTQD_MSASetSpd_kph - KTQD_SetSpdDeltaLong_kph; ...
          | VTQD_MSASetSpd_kph = max (KTQD_MSAActiveMetSpdLo_raw32,VTQD_MSASetSpd_kph);...
          | VTQD_MSASavedSetSpd_kph = VTQD_MSASetSpd_kph;
          | VTQD_DistanceUnit_flg = VINP_Distanceunit_flg
          | %add20230704
          | }
      (junction 298) -> (junction 300) : {VTQD_MSASetSpd_kph = VTQD_MSASetSpd_kph - VTQD_SetSpdDeltaLongFit_kph; ...
          | VTQD_MSASetSpd_kph = max (KTQD_MSAActiveMetSpdLo_raw32,VTQD_MSASetSpd_kph);...
          | VTQD_MSASavedSetSpd_kph = VTQD_MSASetSpd_kph;
          | VTQD_DistanceUnit_flg = VINP_Distanceunit_flg
          | }
          | %add20231127
      (junction 289) -> (junction 291) [order 1] : [VTQD_SetSpdDeltaLongFit_kph  != 0]
      (junction 289) -> (junction 228) [order 2] : %ADD_Long
          | {VTQD_MSASetSpd_kph = VTQD_MSASetSpd_kph + KTQD_SetSpdDeltaLong_kph; ...
          | VTQD_MSASetSpd_kph = min (KTQD_MSAActiveMetSpdHi_raw32,VTQD_MSASetSpd_kph);...
          | VTQD_MSASavedSetSpd_kph = VTQD_MSASetSpd_kph;
          | VTQD_DistanceUnit_flg = VINP_Distanceunit_flg
          | }
      (junction 291) -> (junction 293) : {VTQD_MSASetSpd_kph = VTQD_MSASetSpd_kph + (KTQD_SetSpdDeltaLongFit_kph-VTQD_SetSpdDeltaLongFit_kph); ...
          | VTQD_MSASetSpd_kph = min (KTQD_MSAActiveMetSpdHi_raw32,VTQD_MSASetSpd_kph);...
          | VTQD_MSASavedSetSpd_kph = VTQD_MSASetSpd_kph;
          | VTQD_DistanceUnit_flg = VINP_Distanceunit_flg
          | %add20231127
          | }
    state OFForDisable
      en:
      VTQD_MSASetSpd_kph = 0;
      VTQD_MSASavedSetSpd_kph = VTQD_MSASetSpd_kph;
      VTQD_DistanceUnit_flg = VINP_Distanceunit_flg
    state ACTIVE_or_STANDBY_CHANGE_TO_OFF
      (default) -> (junction 246)
      (junction 246) -> (junction 247) [order 1] : [VTQD_SWCResUpPress_enum == ENUM_SWCBOTTONPRESS_LONGPRESS  ||...
          |  VTQD_SWCResUpPress_enum == ENUM_SWCBOTTONPRESS_SHORTPRESS ||...
          | VTQD_SWCSetDownPress_enum == ENUM_SWCBOTTONPRESS_LONGPRESS  ||...
          |  VTQD_SWCSetDownPress_enum == ENUM_SWCBOTTONPRESS_SHORTPRESS   ]
      (junction 247) -> (junction 248) [order 1] : [VTQD_SWCResUpPress_enum == ENUM_SWCBOTTONPRESS_LONGPRESS  ||...
          |  VTQD_SWCResUpPress_enum == ENUM_SWCBOTTONPRESS_SHORTPRESS]
      (junction 247) -> (junction 250) [order 2] : {VTQD_MSASetSpd_kph = VVMC_MeterIndSpeed_raw32;
          | VTQD_MSASavedSetSpd_kph=VVMC_MeterIndSpeed_raw32;
          | VTQD_MSASetSpd_kph = max (KTQD_MSAActiveMetSpdLo_raw32,VTQD_MSASetSpd_kph);
          | VTQD_MSASavedSetSpd_kph = VTQD_MSASetSpd_kph;;
          | VTQD_DistanceUnit_flg = VINP_Distanceunit_flg
          | }
          | %add20231127
      (junction 248) -> (junction 251) : {VTQD_MSASetSpd_kph = VTQD_MSASavedSetSpd_kph
          | VTQD_MSASavedSetSpd_kph = VTQD_MSASetSpd_kph;;
          | VTQD_DistanceUnit_flg = VINP_Distanceunit_flg}
      (junction 246) -> (junction 249) [order 2]
    state LoopBack
    state SetDown
    (default) -> (junction 188) : {VTQD_DistanceUnit_flg = VINP_Distanceunit_flg}
    (junction 320) -> (junction 307) [order 1] : [VTQD_DistanceUnit_flg == VINP_Distanceunit_flg || VTQD_MSASavedSetSpd_kph <= ONE_FLOAT]
    MSA -> (junction 320)
    (junction 307) -> (junction 188) : {VTQD_MSASetSpd_kph = min (KTQD_MSAActiveMetSpdHi_raw32,VTQD_MSASetSpd_kph);
        | VTQD_MSASavedSetSpd_kph = VTQD_MSASetSpd_kph;}
    (junction 320) -> (junction 306) [order 2]
    (junction 314) -> (junction 307)
    (junction 188) -> (junction 190)
    (junction 306) -> (junction 310) [order 1] : [VINP_Distanceunit_flg == TRUE]
    (junction 306) -> (junction 364) [order 2] : {VTQD_MSASavedSetSpd_kph = (VTQD_MSASavedSetSpd_kph * MPH2KPH)}
    (junction 310) -> (junction 365) : {VTQD_MSASavedSetSpd_kph = (VTQD_MSASavedSetSpd_kph * KPH2MPH)}
    (junction 190) -> (junction 191) [order 1] : [VVMC_MSACrlSta_enum == ENUM_ADASMSASTA_UNDERSPEED ||...
        |  VVMC_MSACrlSta_enum == ENUM_ADASMSASTA_OVERSPEED ||...
        | VVMC_MSACrlSta_enum == ENUM_ADASMSASTA_ERROR ||...
        |  VVMC_MSACrlSta_enum == ENUM_ADASMSASTA_INVAILD  ||...
        |  VVMC_MSACrlSta_enum == ENUM_ADASMSASTA_OFF] %W Add
    (junction 190) -> (junction 192) [order 2]
    (junction 191) -> OFForDisable
    (junction 192) -> (junction 193) [order 1] : [VVMC_MSACrlSta_enum == ENUM_ADASMSASTA_ACTIVE]
        | %W Delete || VINP_MSACrlSta_enum == ENUM_ADASMSASTA_STANDBY]
    (junction 192) -> (junction 194) [order 2]
    (junction 193) -> Active : {VTQD_MSASetSpd_kph = VTQD_MSASavedSetSpd_kph;
        | VTQD_MSASavedSetSpd_kph = VTQD_MSASetSpd_kph;;
        | VTQD_DistanceUnit_flg = VINP_Distanceunit_flg}
    (junction 364) -> (junction 346) [order 1] : [VTQD_MSASavedSetSpd_kph < KTQD_MSAActiveMetSpdLo_kph]
    (junction 365) -> (junction 332) [order 1] : [VTQD_MSASavedSetSpd_kph < KTQD_MSAActiveMetSpdLoMPH_mph]
    (junction 364) -> (junction 348) [order 2]
    (junction 346) -> (junction 345) : {VTQD_MSASavedSetSpd_kph = KTQD_MSAActiveMetSpdLo_kph}
    (junction 365) -> (junction 336) [order 2]
    (junction 332) -> (junction 333) : {VTQD_MSASavedSetSpd_kph = KTQD_MSAActiveMetSpdLoMPH_mph}
    (junction 194) -> (junction 195) [order 1] : [VVMC_MSACrlSta_enum == ENUM_ADASMSASTA_UNLIMIT ||...
        |  VVMC_MSACrlSta_enum == ENUM_ADASMSASTA_STANDBY] %W Add
        |  %W Delete  ||  VINP_MSACrlSta_enum == ENUM_ADASMSASTA_OFF
        | %add 20231127
    (junction 195) -> (junction 196) [order 1] : [VTQD_ChangeToOFF_flg]
    (junction 333) -> (junction 336)
    (junction 345) -> (junction 348)
    (junction 194) -> LoopBack [order 2] : {VTQD_MSASetSpd_kph = VTQD_MSASavedSetSpd_kph;
        | VTQD_MSASavedSetSpd_kph = VTQD_MSASetSpd_kph;;
        | VTQD_DistanceUnit_flg = VINP_Distanceunit_flg}
    (junction 195) -> (junction 197) [order 2]
    (junction 196) -> ACTIVE_or_STANDBY_CHANGE_TO_OFF : {VTQD_MSASetSpd_kph = VTQD_MSASavedSetSpd_kph;
        | VTQD_MSASavedSetSpd_kph = VTQD_MSASetSpd_kph;;
        | VTQD_DistanceUnit_flg = VINP_Distanceunit_flg}
    (junction 336) -> (junction 344)
    (junction 348) -> (junction 354)
    (junction 354) -> (junction 352) [order 1] : [VTQD_MSASavedSetSpd_kph > KTQD_MSAActiveMetSpdHi_kph]
    (junction 344) -> (junction 340) [order 1] : [VTQD_MSASavedSetSpd_kph > KTQD_MSAActiveMetSpdHiMPH_mph]
    (junction 354) -> (junction 357) [order 2]
    (junction 352) -> (junction 353) : {VTQD_MSASavedSetSpd_kph = KTQD_MSAActiveMetSpdHi_kph}
    (junction 344) -> (junction 341) [order 2]
    (junction 340) -> (junction 343) : {VTQD_MSASavedSetSpd_kph = KTQD_MSAActiveMetSpdHiMPH_mph}
    (junction 197) -> (junction 198) [order 1] : [VTQD_SWCSetDownPress_enum == ENUM_SWCBOTTONPRESS_LONGPRESS  ||...
        |  VTQD_SWCSetDownPress_enum == ENUM_SWCBOTTONPRESS_SHORTPRESS  ]
    (junction 197) -> LoopBack [order 2] : {VTQD_MSASetSpd_kph = VTQD_MSASavedSetSpd_kph;
        | VTQD_MSASavedSetSpd_kph = VTQD_MSASetSpd_kph;;
        | VTQD_DistanceUnit_flg = VINP_Distanceunit_flg}
    (junction 198) -> SetDown : {VTQD_MSASetSpd_kph = VVMC_MeterIndSpeed_raw32;
        | VTQD_MSASavedSetSpd_kph=VVMC_MeterIndSpeed_raw32;
        | VTQD_MSASetSpd_kph = max (KTQD_MSAActiveMetSpdLo_raw32,VTQD_MSASetSpd_kph);
        | VTQD_MSASavedSetSpd_kph = VTQD_MSASetSpd_kph;;
        | VTQD_DistanceUnit_flg = VINP_Distanceunit_flg}
        | %add20231118
    (junction 353) -> (junction 357)
    (junction 343) -> (junction 341)
    (junction 357) -> (junction 312)
    (junction 341) -> (junction 311)
    (junction 312) -> (junction 311)
    (junction 311) -> (junction 314)
  data: KTQD_SetSpdDeltaLong_kph input; KTQD_SetSpdDeltaShort_kph input; VTQD_SWCSetDownPress_enum input; VINP_Distanceunit_flg input; VTQD_ChangeToOFF_flg input; VVMC_MeterIndSpeed_raw32 input; KTQD_MSAActiveMetSpdHi_raw32 input; KTQD_MSAActiveMetSpdLo_raw32 input; VVMC_MSACrlSta_enum input; VTQD_SetSpdDeltaLongFit_kph input; KTQD_SetSpdDeltaLongFit_kph input; VTQD_MSASavedSetSpd_kph local double; ENUM_ADASMSASTA_ACTIVE parameter; ENUM_ADASMSASTA_ERROR parameter; ENUM_ADASMSASTA_INVAILD parameter; ENUM_ADASMSASTA_OFF parameter; ENUM_ADASMSASTA_OVERSPEED parameter; ENUM_ADASMSASTA_STANDBY parameter; ENUM_ADASMSASTA_UNDERSPEED parameter; VTQD_MSASetSpd_kph output single; ENUM_SWCBOTTONPRESS_LONGPRESS parameter; ENUM_SWCBOTTONPRESS_SHORTPRESS parameter; VTQD_SWCResUpPress_enum input; ENUM_ADASMSASTA_UNLIMIT parameter; KPH2MPH parameter; MPH2KPH parameter; TRUE parameter; VTQD_DistanceUnit_flg local boolean; ONE_FLOAT parameter; KTQD_MSAActiveMetSpdHiMPH_mph parameter; KTQD_MSAActiveMetSpdLoMPH_mph parameter; KTQD_MSAActiveMetSpdLo_kph parameter; KTQD_MSAActiveMetSpdHi_kph parameter

== stateflow chart tqdtqr_rebuild_V3/Input_Convert/Signal function/SWC1 SWC2 status/SWC_Subsystem/Speed Setting Mode/MSA Speed Setting ON/Specific_STATE_ChangeToOFF ==
  state FLG_ON
    en:
    VTQD_ChangeToOFF_flg = TRUE;
  state Initialize
    en:
    VTQD_ChangeToOFF_flg = FALSE;
  state STAY
  (default) -> Initialize
  Initialize -> STAY : [VINP_MSACrlSta_enum == ENUM_ADASMSASTA_UNLIMIT ||...
      | VINP_MSACrlSta_enum == ENUM_ADASMSASTA_ACTIVE]
  STAY -> FLG_ON [order 1] : [VINP_MSACrlSta_enum == ENUM_ADASMSASTA_STANDBY]
  STAY -> Initialize [order 2] : [VINP_MSACrlSta_enum != ENUM_ADASMSASTA_STANDBY &&...
      | VINP_MSACrlSta_enum != ENUM_ADASMSASTA_ACTIVE&&...
      | VINP_MSACrlSta_enum != ENUM_ADASMSASTA_UNLIMIT]
  (junction 11) -> Initialize
  FLG_ON -> (junction 9)
  (junction 9) -> (junction 11) : [VINP_MSACrlSta_enum != ENUM_ADASMSASTA_STANDBY]
  data: VINP_MSACrlSta_enum input; VTQD_ChangeToOFF_flg output boolean; FALSE parameter; TRUE parameter; ENUM_ADASMSASTA_ACTIVE parameter; ENUM_ADASMSASTA_STANDBY parameter; ENUM_ADASMSASTA_UNLIMIT parameter
